simulink model "Induction_Generator_modeling"  (R2016a)
settings: Solver=VariableStepAuto  StartTime=0.0  StopTime=1  MaxStep=1e-4  RelTol=1e-3
libraries: powerlib x9
settings Model: Creator=AT Once  LastModifiedBy=AT Once

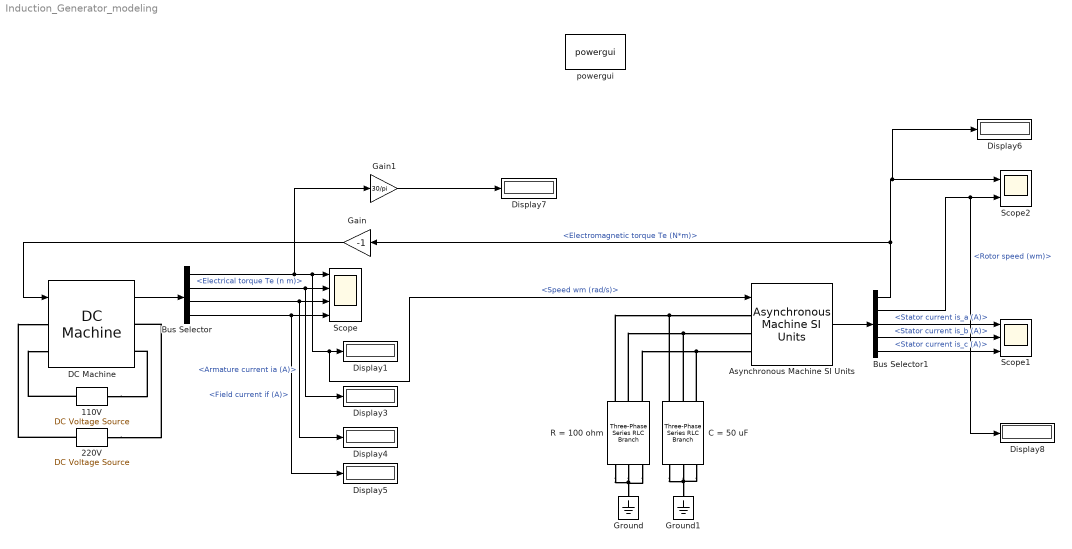
== system Induction_Generator_modeling ==
  110V : powerlib/Electrical Sources/DC Voltage Source  Amplitude=100  Measurements=None
  220V : powerlib/Electrical Sources/DC Voltage Source  Amplitude=220  Measurements=None
  Asynchronous Machine SI Units : powerlib/Machines/Asynchronous Machine SI Units  RotorType=Squirrel-cage  PresetModel=No  MechanicalLoad=Speed w  ShowDetailedParameters=on  ReferenceFrame=Stationary  Units=SI  MeasurementBus=off  NominalParameters=[2.2e+3 380 50]  Stator=[2.1484 9e-3]  Rotor=[2.831 9e-3]  Cage1=[0.4155 0.002066]  Cage2=[0.4168 0.0003495]  Lm=0.1318  Mechanical=[0.05 0.005879 2]  PolePairs=2  InitialConditions=[1 0 1 1 1 0 -120 120]  SimulateSaturation=off  Saturation=[14.03593122, 27.81365428, 53.79336849, 72.68890987, 97.98006896, 148.6815601, 215.7428561, 302.9841135, 428.7778367 ; 230, 322, 414, 460, 506, 552, 598, 644, 690]  LoadFlowParameters=1492000  TsPowergui=0  TsBlock=-1  IterativeModel=Trapezoidal non iterative  IterativeDiscreteModel=Trapezoidal non iterative  Pmec=0
  Bus Selector : BusSelector  OutputSignals=Speed wm (rad/s),Electrical torque Te (n m),Armature current ia (A),Field current if (A)
  Bus Selector1 : BusSelector  OutputSignals=Mechanical.Electromagnetic torque Te (N*m),Mechanical.Rotor speed (wm),Stator measurements.Stator current is_a (A),Stator measurements.Stator current is_b (A),Stator measurements.Stator current is_c (A)
  C = 50 uF : powerlib/Elements/Three-Phase Series RLC Branch  LConnTagsString=A|B|C  RConnTagsString=A|B|C  BranchType=C  Resistance=1  Inductance=1e-3  Capacitance=1e-6  Measurements=None
  DC Machine : powerlib/Machines/DC Machine  PresetModel=No  MechanicalLoad=Torque TL  FieldType=Wound  ShowDetailedParameters=on  MeasurementBus=off  RLa=[1.45 0.2]  RLf=[110/0.4 0.5]  Laf=1.8  MachineConstant=Torque constant (N.m/A)  Ke=1.8  Kt=1.8  J=0.02215  Bm=0.002953  Tf=0.5161  w0=0  Ifinit=0  TsPowergui=0  TsBlock=-1
  Display{1,3..8} (7 alike) : Display
  Gain : Gain  Gain=-1
  Gain1 : Gain  Gain=30/pi
  Ground : powerlib/Elements/Ground  LConnTagsString=a
  Ground1 : powerlib/Elements/Ground  LConnTagsString=a
  R = 100 ohm : powerlib/Elements/Three-Phase Series RLC Branch  LConnTagsString=A|B|C  RConnTagsString=A|B|C  BranchType=R  Resistance=1  Inductance=1e-3  Capacitance=1e-6  Measurements=None
  Scope : Scope  NumInputPorts=4
  Scope1 : Scope  NumInputPorts=3
  Scope2 : Scope  NumInputPorts=2
  powergui : powerlib/powergui  Priority=1  SimulationMode=Continuous  SolverType=Tustin/Backward Euler (TBE)  SampleTime=50e-6  frequency=60  SPID=off  DisableSnubberDevices=off  DisableRonSwitches=off  DisableVfSwitches=off  SwTol=0  DisplayEquations=off  Interpol=off  ExternalGateDelay=off  methode=off  Ts=10  FunctionMessages=off  echomessages=off  HookPort=off  EnableUseOfTLC=off  x0status=blocks  frequencyindice=50  Pbase=100e6  ErrMax=1e-4  Iterations=50  UnitsV=kV  UnitsW=MW  buscounter=0  RestoreLinks=warning  ResistiveCurrentMeasurement=off  Frange=[0:2:500]  Ylog=off  Xlog=on  ShowGrid=off  save=off  variable=ZData  structure=0  ZoomFFT=off  StartTime=0.0  cycles=1  DisplayStyle=1  fundamental=60  FreqAxis=off  MaxFrequency=1000  frequencyindicesteady=1  RmsSteady=1  display=off
  wires:
  DC Machine/1 -> Bus Selector/1
  Bus Selector/4 -> Scope/4, Display5/1  "<Field current if (A)>"
  Bus Selector/3 -> Display4/1, Scope/3  "<Armature current ia (A)>"
  Bus Selector/2 -> Scope/2, Display3/1  "<Electrical torque Te (n m)>"
  Bus Selector/1 -> Gain1/1, Scope/1, Asynchronous Machine SI Units/1, Display1/1  "<Speed wm (rad/s)>"
  Asynchronous Machine SI Units/1 -> Bus Selector1/1
  Bus Selector1/1 -> Display6/1, Scope2/1, Gain/1  "<Electromagnetic torque Te (N*m)>"
  Gain/1 -> DC Machine/1
  Bus Selector1/3 -> Scope1/1  "<Stator current is_a (A)>"
  Bus Selector1/4 -> Scope1/2  "<Stator current is_b (A)>"
  Bus Selector1/5 -> Scope1/3  "<Stator current is_c (A)>"
  Bus Selector1/2 -> Display8/1, Scope2/2  "<Rotor speed (wm)>"
  Gain1/1 -> Display7/1
  connections:
  R = 100 ohm/RConn1 -- R = 100 ohm/RConn2 -- Ground/LConn1 -- R = 100 ohm/RConn3
  C = 50 uF/RConn1 -- C = 50 uF/RConn2 -- C = 50 uF/RConn3 -- Ground1/LConn1
  220V/LConn1 -- DC Machine/RConn1
  220V/RConn1 -- DC Machine/LConn1
  110V/LConn1 -- DC Machine/RConn2
  110V/RConn1 -- DC Machine/LConn2
  C = 50 uF/LConn1 -- R = 100 ohm/LConn1 -- Asynchronous Machine SI Units/LConn1
  C = 50 uF/LConn2 -- Asynchronous Machine SI Units/LConn2 -- R = 100 ohm/LConn2
  C = 50 uF/LConn3 -- Asynchronous Machine SI Units/LConn3 -- R = 100 ohm/LConn3
